simulink model "EmergencyNetwork"  (R2026b)
settings: Solver=FixedStepDiscrete  StopTime=49  FixedStep=1
values from neighbouring files (symbols this model uses):
  nodePositions = [137.273050427 -4.6533338035 10]    [gcs_survey_data.mat]    (also in setupGCS.m = zeros(numNodes, 3); setupPhase1.m = [150 200 10)
settings Model: Creator=RonieSamuel  LastModifiedBy=test

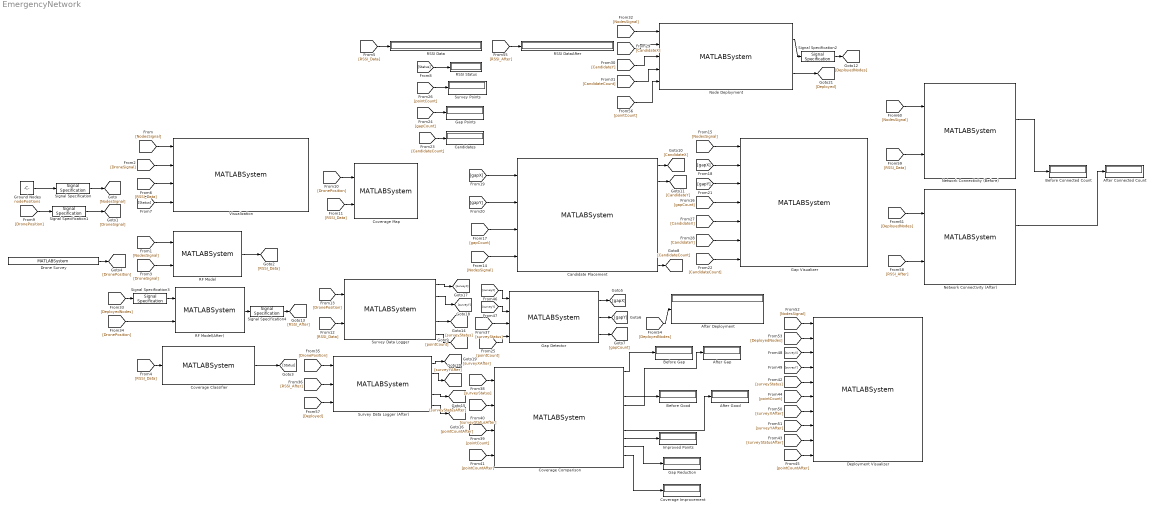
== system EmergencyNetwork ==
  After Connected Count : Display
  After Deployment : Display
  After Gap : Display
  After Good : Display
  Before Connected Count : Display
  Before Gap : Display
  Before Good : Display
  Candidate Placement : MATLABSystem  System=CandidatePlacement  GapClusterDistance=250  MaxPoints=25  MaxCandidates=25  SurveyAltitude=30  AreaSize=[ 1000, 1000 ]  Buildings=[]  GapCountWeight=10  DistanceWeight=0.1  RFRangeScale=0.25  SimulateUsing=Interpreted execution
      mask Type: CandidatePlacement
  Candidates : Display
  Coverage Classifier : MATLABSystem  System=CoverageClassifier  GoodThreshold=-60  ModerateThreshold=-75  WeakThreshold=-85  SimulateUsing=Interpreted execution
      mask Type: CoverageClassifier
  Coverage Comparison : MATLABSystem  System=CoverageComparison  MaxPoints=25  SimulateUsing=Interpreted execution
      mask Type: CoverageComparison
  Coverage Improvement : Display
  Coverage Map : MATLABSystem  System=CoverageMap  AreaSize=[ 1000, 1000 ]  MaxPoints=25  SimulateUsing=Interpreted execution
      mask Type: CoverageMap
  Deployment Visualizer : MATLABSystem  System=DeploymentVisualizer  AreaSize=[ 1000, 1000 ]  Buildings=[]  SimulateUsing=Interpreted execution
      mask Type: DeploymentVisualizer
  Drone Survey : MATLABSystem  System=DroneSurvey  SurveyPoints=[ 50, 50, 30; 250, 50, 30; 450, 50, 30; 650, 50, 30; 850, 50, 30; 850, 250, 30; 650, 250, 30; 450, 250, 30; 250, 250, 30; 50, 250, 30; 50, 450, 30; 250, 450, 30; 450, 450, 30; 650, 450, 30; 850, 450, 30; 850, 650, 30; 650, 650, 30; 450, 650, 30; 250, 650, 30; 50, 650, 30; 50, 850, 30; 250, 850, 30; 450, 850, 30; 650, 850, 30; 850, 850, 30 ]  SimulateUsing=Interpreted execution
      mask Type: DroneSurvey
  Gap Detector : MATLABSystem  System=GapDetector  MaxPoints=25  SimulateUsing=Interpreted execution
      mask Type: GapDetector
  Gap Points : Display
  Gap Reduction : Display
  Gap Visualizer : MATLABSystem  System=GapVisualizer  AreaSize=[ 1000, 1000 ]  Buildings=[]  SimulateUsing=Interpreted execution
      mask Type: GapVisualizer
  Ground Nodes : Constant  Value=nodePositions  VectorParams1D=off
  Improved Points : Display
  Network Connectivity (After) : MATLABSystem  System=NetworkConnectivity  CommunicationThreshold=-85  SimulateUsing=Code generation
      mask Type: NetworkConnectivity
  Network Connectivity (Before) : MATLABSystem  System=NetworkConnectivity  CommunicationThreshold=-85  SimulateUsing=Code generation
      mask Type: NetworkConnectivity
  Node Deployment : MATLABSystem  System=NodeDeployment  NewNodeAltitude=10  MaxPoints=25  SimulateUsing=Interpreted execution
      mask Type: NodeDeployment
  RF Model : MATLABSystem  System=RFModel  ReferenceRSSI=-30  PathLossExponent=2.2  ReferenceDistance=1  RFRangeScale=0.25  SimulateUsing=Interpreted execution
      mask Type: RFModel
  RF Model(After) : MATLABSystem  System=RFModel  ReferenceRSSI=-30  PathLossExponent=2.2  ReferenceDistance=1  RFRangeScale=0.25  SimulateUsing=Interpreted execution
      mask Type: RFModel
  RSSI Data : Display
  RSSI DataAfter : Display
  RSSI Status : Display
  Signal Specification : SignalSpecification  Dimensions=[3 3]
  Signal Specification1 : SignalSpecification  Dimensions=[1 3]
  Signal Specification2 : SignalSpecification  Dimensions=[4 3]
  Signal Specification3 : SignalSpecification  Dimensions=[4,3]
  Signal Specification4 : SignalSpecification  Dimensions=[1,4]
  Survey Data Logger : MATLABSystem  System=SurveyDataLogger  MaxPoints=25  SimulateUsing=Interpreted execution
      mask Type: SurveyDataLogger
  Survey Data Logger (After) : MATLABSystem  System=SurveyDataLoggerAfter  MaxPoints=25  SimulateUsing=Interpreted execution
      mask Type: SurveyDataLoggerAfter
  Survey Points : Display
  Visualization : MATLABSystem  System=EnvironmentVisualizer  AreaSize=areaSize  NodeLabels=nodeLabels  Buildings=buildings  SimulateUsing=Interpreted execution
      mask Type: EnvironmentVisualizer
  wires:
  Ground Nodes/1 -> Signal Specification/1
  Signal Specification/1 -> [NodesSignal]
  [NodesSignal] -> Visualization/1
  [NodesSignal] -> RF Model/1
  Signal Specification1/1 -> [DroneSignal]
  [DroneSignal] -> Visualization/2
  [DroneSignal] -> RF Model/2
  RF Model/1 -> [RSSI_Data]
  [RSSI_Data] -> RSSI Data/1
  [RSSI_Data] -> Visualization/3
  Coverage Classifier/1 -> [Status]
  [Status] -> Visualization/4
  [Status] -> RSSI Status/1
  [RSSI_Data] -> Coverage Classifier/1
  Drone Survey/1 -> [DronePosition]
  [DronePosition] -> Signal Specification1/1
  [DronePosition] -> Coverage Map/1
  [RSSI_Data] -> Coverage Map/2
  [RSSI_Data] -> Survey Data Logger/2
  [DronePosition] -> Survey Data Logger/1
  [NodesSignal] -> Candidate Placement/4
  [NodesSignal] -> Gap Visualizer/1
  Gap Detector/1 -> [gapX]
  Gap Detector/2 -> [gapY]
  Gap Detector/3 -> [gapCount]
  [gapCount] -> Candidate Placement/3
  [gapY] -> Candidate Placement/2
  [gapX] -> Candidate Placement/1
  [gapX] -> Gap Visualizer/2
  [gapY] -> Gap Visualizer/3
  [gapCount] -> Gap Visualizer/4
  Candidate Placement/7 -> [CandidateCount]
  [CandidateCount] -> Gap Visualizer/7
  [CandidateCount] -> Candidates/1
  [gapCount] -> Gap Points/1
  Survey Data Logger/5 -> [pointCount]
  [pointCount] -> Gap Detector/4
  [pointCount] -> Survey Points/1
  Candidate Placement/1 -> [CandidateX]
  Candidate Placement/2 -> [CandidateY]
  [CandidateX] -> Gap Visualizer/5
  [CandidateY] -> Gap Visualizer/6
  [CandidateY] -> Node Deployment/3
  [CandidateX] -> Node Deployment/2
  [CandidateCount] -> Node Deployment/4
  [NodesSignal] -> Node Deployment/1
  Signal Specification2/1 -> [DeployedNodes]
  Node Deployment/1 -> Signal Specification2/1
  [DeployedNodes] -> Signal Specification3/1
  Signal Specification3/1 -> RF Model(After)/1
  [DronePosition] -> RF Model(After)/2
  RF Model(After)/1 -> Signal Specification4/1
  Signal Specification4/1 -> [RSSI_After]
  Survey Data Logger/4 -> [surveyStatus]
  [surveyStatus] -> Gap Detector/3
  [surveyStatus] -> Coverage Comparison/1
  [pointCount] -> Coverage Comparison/3
  [surveyStatusAfter] -> Coverage Comparison/2
  [pointCountAfter] -> Coverage Comparison/4
  [surveyStatus] -> Deployment Visualizer/5
  [surveyStatusAfter] -> Deployment Visualizer/9
  [pointCount] -> Deployment Visualizer/6
  [pointCountAfter] -> Deployment Visualizer/10
  Survey Data Logger/1 -> [surveyX]
  Survey Data Logger/2 -> [surveyY]
  [surveyY] -> Gap Detector/2
  [surveyX] -> Gap Detector/1
  [surveyY] -> Deployment Visualizer/4
  [surveyX] -> Deployment Visualizer/3
  [surveyXAfter] -> Deployment Visualizer/7
  [surveyYAfter] -> Deployment Visualizer/8
  [DeployedNodes] -> Deployment Visualizer/2
  [NodesSignal] -> Deployment Visualizer/1
  Coverage Comparison/1 -> Before Gap/1
  Coverage Comparison/5 -> After Gap/1
  Coverage Comparison/4 -> Before Good/1
  Coverage Comparison/8 -> After Good/1
  Coverage Comparison/9 -> Improved Points/1
  Coverage Comparison/10 -> Gap Reduction/1
  Coverage Comparison/11 -> Coverage Improvement/1
  [DeployedNodes] -> After Deployment/1
  [RSSI_After] -> RSSI DataAfter/1
  [pointCount] -> Node Deployment/5
  [DronePosition] -> Survey Data Logger (After)/1
  [RSSI_After] -> Survey Data Logger (After)/2
  Node Deployment/2 -> [Deployed]
  [Deployed] -> Survey Data Logger (After)/3
  Survey Data Logger (After)/1 -> [surveyXAfter]
  Survey Data Logger (After)/2 -> [surveyYAfter]
  Survey Data Logger (After)/5 -> [pointCountAfter]
  Survey Data Logger (After)/4 -> [surveyStatusAfter]
  [RSSI_Data] -> Network Connectivity (Before)/2
  [RSSI_After] -> Network Connectivity (After)/2
  [NodesSignal] -> Network Connectivity (Before)/1
  [DeployedNodes] -> Network Connectivity (After)/1
  Network Connectivity (Before)/2 -> Before Connected Count/1
  Network Connectivity (After)/2 -> After Connected Count/1
